simulink model "EVTOLTiltrotor"  (R2024b)
settings: Solver=ode1  StartTime=0.0  StopTime=simTime  RelTol=1e-3  AbsTol=1e-3
undefined symbols (not defined in the file): battery, CityMission, control, FixedWingMission, flightState, FSState, HoverMission, iniRoll, initPitch, iniYaw, params, percWeightGain, position, R_LOOKAHEAD, tiltIni, TransitionMission, uavParam, UAVSampleTime, vIni, Vt, xGround, yGround, zGround
libraries: uavalgslib x7, simulink x4, sharedtransform x2, shared6dof x1, simulink_extras x1, sim3dlib x1, uavsim3dlib x1, uavutilslib x1
(part 1 of 2)
settings Model: DataDictionary=VTOLDynamicsData.sldd  PauseTimes=2  Creator=jjha  LastModifiedBy=jjha
settings SolverCC: AutoInsertRateTranBlk=on  DecoupledContinuousIntegration=on
settings RTWCC: GPUComputeCapability=3.5

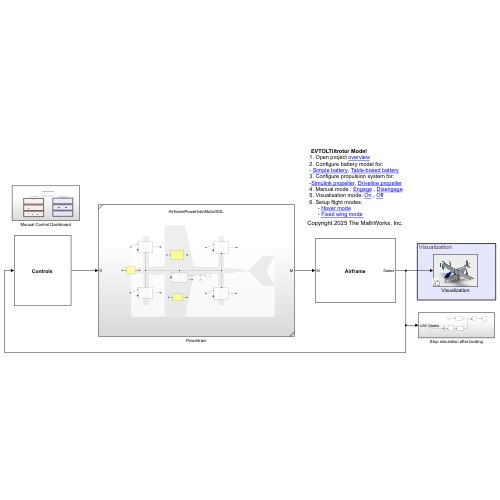
[thumbnail: Simulink's stored preview of the top-level diagram]
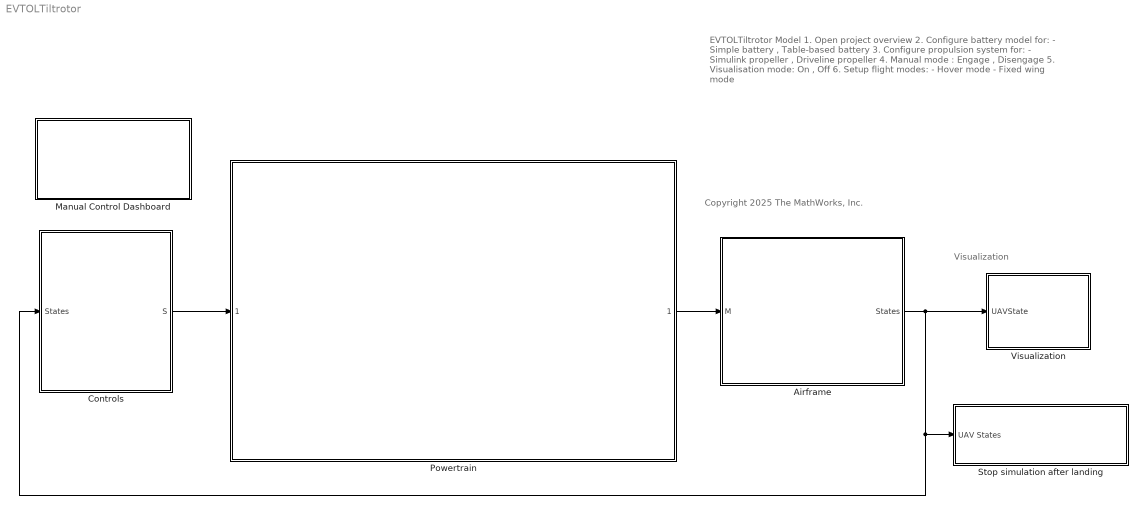
== system EVTOLTiltrotor ==
  note: Copyright 2025 The MathWorks, Inc.
  note: Visualization
  note: EVTOLTiltrotor Model
      | 1. Open project overview
      | 2. Configure battery model for:
      | - Simple battery , Table-based battery
      | 3. Configure propulsion system for:
      | - Simulink propeller , Driveline propeller
      | 4. Manual mode : Engage , Disengage
      | 5. Visualisation mode: On , Off
      | 6. Setup flight modes:
      | - Hover mode
      | - Fixed wing mode
  Airframe : Subsystem
      mask Display:
      | %disp(get_param(gcb, 'Name'))
      | disp(['{\bf\fontsize{12}' get_param(gcb, 'Name') '}'], 'texmode','on');
  Controls : Subsystem
      mask Display:
      | %disp(get_param(gcb, 'Name'))
      | disp(['{\bf\fontsize{12}' get_param(gcb, 'Name') '}'], 'texmode','on');
  Manual Control Dashboard : Subsystem
  Powertrain : Subsystem  ReferencedSubsystem=AirframePowertrainMotorSDL
  Stop simulation after landing : Subsystem
  Visualization : Subsystem  Variant=on  VariantControl=Visualization
      mask Display: image('TiltrotorVisualization.PNG'); % Use "Edit Image" on toolstrip to change.
  wires:
  Controls/1(S) -> Powertrain/1
  Airframe/1(States) -> Controls/1(States), Stop simulation after landing/1(UAV States), Visualization/1(UAVState)
  Powertrain/1 -> Airframe/1(M)

== system EVTOLTiltrotor/Airframe ==
  M : Inport
  6DOF (Euler Angles) : shared6dof/6DOF (Euler Angles)  units=Metric (MKS)  mtype=Fixed  rep=Euler Angles  xme_0=[xGround, yGround, zGround]  Vm_0=[vIni 0 0]  eul_0=[iniRoll initPitch iniYaw]  pm_0=[0 0 0]  mass_0=6.031*percWeightGain  mass_e=0.5  mass_f=2.0  inertia=[uavParam.geom.Ixx 0 0; 0 uavParam.geom.Iyy 0; 0 0 uavParam.geom.Izz]*percWeightGain  inertia_e=eye(3)  inertia_f=2*eye(3)  k_quat=1.0  vre_flag=on  abi_flag=on  aMode=0  xme_statename=''  Vm_statename=''  eul_statename=''  quat_statename=''  pm_statename=''  mass_statename=''
  Energy : Subsystem
      mask Display:
      | %disp(get_param(gcb, 'Name'))
      | disp(['{\bf\fontsize{12}' get_param(gcb, 'Name') '}'], 'texmode','on');
  Ground Truth Bus : Subsystem
  Input : Subsystem
  Scope : Scope  NumInputPorts=2
  Terminator : Terminator
  States : Outport
  wires:
  Input/4(AirData) -> Ground Truth Bus/10(AirData)
  Input/3(RotorPar) -> Ground Truth Bus/9(RotorParams)
  Ground Truth Bus/1(Ground Truth) -> States/1  "States"
  Input/2(M) -> Scope/2, 6DOF (Euler Angles)/2  "Moment"
  Input/1(F) -> Scope/1, 6DOF (Euler Angles)/1  "Thrust"
  6DOF (Euler Angles)/9 -> Ground Truth Bus/8(Abe)
  6DOF (Euler Angles)/7 -> Terminator/1
  6DOF (Euler Angles)/8 -> Ground Truth Bus/7(Abb)  "Abb"
  6DOF (Euler Angles)/5 -> Ground Truth Bus/5(Vb)  "Vb"
  6DOF (Euler Angles)/1 -> Ground Truth Bus/1(Ve)  "Ve"
  6DOF (Euler Angles)/2 -> Ground Truth Bus/2(Xe)  "Xe"
  6DOF (Euler Angles)/4 -> Ground Truth Bus/4(DCMbe)  "DCMbe"
  6DOF (Euler Angles)/3 -> Ground Truth Bus/3(Euler)  "Euler"
  6DOF (Euler Angles)/6 -> Ground Truth Bus/6(pqr)  "pqr"
  M/1 -> Energy/1(s), Input/1(m)

== system EVTOLTiltrotor/Controls ==
  States : Inport
  Bus Creator : BusCreator  Inputs=2
  Constant1 : Constant
  Flight Control : Subsystem  ReferencedSubsystem=FlightControl
      settings: PortSchema="{\"entries\":[{\"content\":{\"sides\":[{\"content\":{\"connectorIds\":[\"In1\",\"In3\",\"In2\"]},\"type\":\"ConnectorPlacement.EquallySpacedRectSide\",\"uuid\":\"16133643-a271-41ca-af0b-35692e75911e\"},{\"content\":{\"connectorIds\":[\"Out1\",\"Out3\",\"Out2\"],\"side\":\"RIGHT\"},\"type\":\"ConnectorPlacement.EquallySpacedRectSide\",\"uuid\":\"71f512ce-dc43-4a94-9ca9-7a68bb7e8691\"},{\"content\":{\"side\":\"TOP\"},\"type\":\"ConnectorPlacement.EquallySpacedRectSide\",\"uuid\":\"92fc6d85-868c-4302-9641-f62c34b61a8f\"}]},\"type\":\"ConnectorPlacement.EquallySpacedConnector\",\"uuid\":\"8e64feec-9c48-46d7-b9b5-e6a25dfded6a\"}],\"packageUris\":[\"http://schema.mathworks.com/mf0/Connector/R2020b\"],\"version\":\"1.0\"}"
  Guidance Test Bench : Subsystem
  Output : Subsystem
  Sensor : Subsystem
  noQGC : Subsystem  TreatAsAtomicUnit=on  SystemSampleTime=UAVSampleTime*4  VariantControl=useQGC==0
  S : Outport
  wires:
  Output/1(S) -> S/1
  Bus Creator/1 -> Output/1(Act)
  Flight Control/3 -> Bus Creator/2  "Tq"
  Flight Control/1 -> Bus Creator/1  "Actuator"
  noQGC/1(Mission) -> Guidance Test Bench/1(Global Mission)
  Guidance Test Bench/1(Cmd) -> Flight Control/1
  States/1 -> Output/3(States), Sensor/1("  "), Guidance Test Bench/2(Aircraft States)
  Flight Control/2 -> Output/2(Ctrl)  "CtrlSurfaces"
  Sensor/1(" ") -> Flight Control/2
  Constant1/1 -> Flight Control/3

== system EVTOLTiltrotor/Manual Control Dashboard ==
  note: Commanded Altitude
  note: Flight Mode
  note: Commanded Y (m)
  note: Fixed Wing
  note: Commanded Airspeed (m)
  note: Hover
  note: Transition
  note: Commanded Course
  note: Fixed Wing Commands
  note: Hover Commands
  note: Commanded Altitude (m)
  note: Back Transition
  note: Commanded X (m)
  note: Change these parameters during simulation when using manual testbench mode. To engage manual testbench mode set variable TestMode=0
  FlightModeSlider : SliderBlock  LabelPosition=Hide  ScaleMax=3  TickInterval=1
  Slider1 : SliderBlock  LabelPosition=Hide  ScaleMax=50  TickInterval=5
  Slider2 : SliderBlock  LabelPosition=Hide  ScaleMin=-30  ScaleMax=30  TickInterval=5
  Slider3 : SliderBlock  LabelPosition=Hide  ScaleMin=-30  ScaleMax=30  TickInterval=5
  Slider5 : SliderBlock  LabelPosition=Hide  ScaleMin=-30  ScaleMax=30  TickInterval=5
  Slider6 : SliderBlock  LabelPosition=Hide  ScaleMin=-100  TickInterval=10
  Slider7 : SliderBlock  LabelPosition=Hide  ScaleMin=10  ScaleMax=30  TickInterval=5

== system EVTOLTiltrotor/Stop simulation after landing ==
  UAV States : Inport
  AND : Logic  IconShape=distinctive  AllPortsSameDT=off  OutDataTypeStr=boolean
  Bus Selector : BusSelector  OutputSignals=Xe
  Clock : Clock
  Compare To Constant : simulink/Logic and Bit Operations/Compare To Constant  relop=>=  const=-1e-1  OutDataTypeStr=boolean
  Compare To Constant1 : simulink/Logic and Bit Operations/Compare To Constant  relop=>=  const=5  OutDataTypeStr=boolean
  Selector : Selector  InputPortWidth=3  IndexOptions=Index vector (dialog)  Indices=3  OutputSizes=1
  Stop Simulation : Stop
  wires:
  Bus Selector/1 -> Selector/1  "<Xe>"
  AND/1 -> Stop Simulation/1
  Compare To Constant1/1 -> AND/1
  UAV States/1 -> Bus Selector/1
  Clock/1 -> Compare To Constant1/1
  Compare To Constant/1 -> AND/2
  Selector/1 -> Compare To Constant/1

== system EVTOLTiltrotor/Visualization ==
  UAVState : Inport
  No Visualization : Subsystem  VariantControl=Visualization==0
  Photorealistic : Subsystem  VariantControl=Visualization==2
  Visualization : Subsystem  VariantControl=Visualization==1

== system EVTOLTiltrotor/Airframe/Energy ==
  note: Range Estimator
  s : Inport
  Add : Sum  Inputs=++++
  Add1 : Sum
  Bus Selector : BusSelector  OutputSignals=R1.Info,R2.Info,R3.Info,R4.Info,A.AirData.airspeed,Batt.Current,Batt.Volt
  Distance : Subsystem
  Energy : Display
  Energy Consumed : Display
  Energy Motor1 : Subsystem
  Energy Motor2 : Subsystem
  Energy Motor3 : Subsystem
  Energy Motor4 : Subsystem
  Online Range : Subsystem
  Range Rating : Subsystem
  Scope : Scope  NumInputPorts=2
  Terminator : Terminator
  Zero division protection : Constant  Value=0.01
  wires:
  Bus Selector/1 -> Energy Motor1/1(M1)  "<Info>"
  Bus Selector/2 -> Energy Motor2/1(M2)  "<Info>"
  Bus Selector/3 -> Energy Motor3/1(M3)  "<Info>"
  Bus Selector/4 -> Energy Motor4/1(M4)  "<Info>"
  Energy Motor2/1(E2) -> Add/2
  Energy Motor3/1(E3) -> Add/3
  Energy Motor4/1(E4) -> Add/4
  Add/1 -> Energy Consumed/1
  Energy Motor1/1(E1) -> Add/1
  Distance/1(Dist) -> Add1/2
  Add1/1 -> Range Rating/1(d)
  Distance/2(SimTime(s)) -> Terminator/1
  Zero division protection/1 -> Add1/1
  Online Range/1(E) -> Range Rating/2(E), Energy/1
  s/1 -> Bus Selector/1
  Bus Selector/5 -> Distance/1(VehSpd)  "<airspeed>"
  Bus Selector/6 -> Scope/1, Online Range/1(I)  "<Current>"
  Bus Selector/7 -> Online Range/2(V), Scope/2  "<Volt>"

== system EVTOLTiltrotor/Airframe/Ground Truth Bus ==
  Ve : Inport
  Xe : Inport  Port=2
  Euler : Inport  Port=3
  DCMbe : Inport  Port=4
  Vb : Inport  Port=5
  pqr : Inport  Port=6
  Abb : Inport  Port=7
  Abe : Inport  Port=8
  RotorParams : Inport  Port=9
  AirData : Inport  Port=10
  Bus Creator : BusCreator  Inputs=13
  Bus Selector : BusSelector  OutputSignals=airspeed
  Direction Cosine Matrix to Quaternions : sharedtransform/Direction Cosine Matrix  to Quaternions  aMode=0  action=None  tolerance=eps(2)
      settings: LibrarySourceBlock=|
      | aerolibtransform2/Direction Cosine Matrix
      | to Quaternions
  Ground Track : MATLAB Function  TreatAsAtomicUnit=on
  To Workspace : ToWorkspace  VariableName=PositionPlotData  SaveFormat=Timeseries  SampleTime=-1
  Ground Truth : Outport
  wires:
  Ve/1 -> Bus Creator/1, Ground Track/1(vxyz)
  Ground Track/1(course) -> Bus Creator/12  "course"
  Ground Track/2(gndSpeed) -> Bus Creator/13  "gndspeed"
  Abe/1 -> Bus Creator/11  "Abe"
  RotorParams/1 -> Bus Creator/8  "RotorParameters"
  Direction Cosine Matrix to Quaternions/1 -> Bus Creator/10  "q"
  Bus Selector/1 -> Bus Creator/9  "<airspeed>"
  AirData/1 -> Bus Selector/1
  Abb/1 -> Bus Creator/7
  Vb/1 -> Bus Creator/5
  Euler/1 -> Bus Creator/3
  DCMbe/1 -> Bus Creator/4, Direction Cosine Matrix to Quaternions/1
  Bus Creator/1 -> Ground Truth/1
  Xe/1 -> To Workspace/1, Bus Creator/2
  pqr/1 -> Bus Creator/6

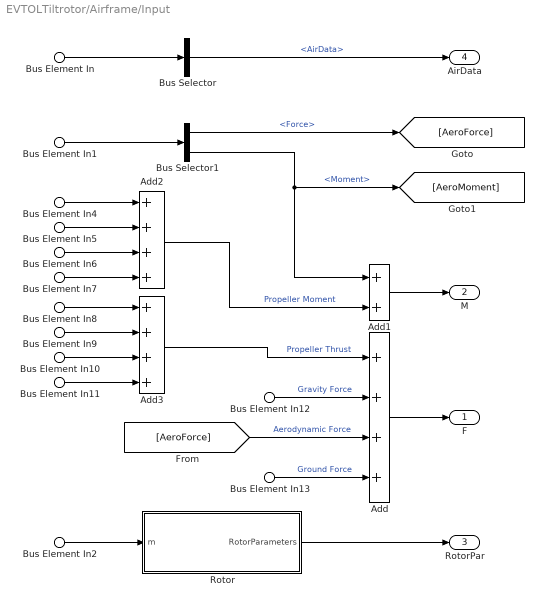
== system EVTOLTiltrotor/Airframe/Input ==
  Bus Element In2 : Inport  PortName=m
  Bus Element In : Inport  PortName=m  Element=A
  Bus Element In1 : Inport  PortName=m  Element=A
  Bus Element In4 : Inport  PortName=m  Element=R1.M
  Bus Element In8 : Inport  PortName=m  Element=R1.F
  Bus Element In5 : Inport  PortName=m  Element=R2.M
  Bus Element In9 : Inport  PortName=m  Element=R2.F
  Bus Element In6 : Inport  PortName=m  Element=R3.M
  Bus Element In10 : Inport  PortName=m  Element=R3.F
  Bus Element In7 : Inport  PortName=m  Element=R4.M
  Bus Element In11 : Inport  PortName=m  Element=R4.F
  Bus Element In12 : Inport  PortName=m  Element=G.gravityForce
  Bus Element In13 : Inport  PortName=m  Element=AD.GroundForce
  Add : Sum  Inputs=++++
  Add1 : Sum
  Add2 : Sum  Inputs=++++
  Add3 : Sum  Inputs=++++
  Bus Selector : BusSelector  OutputSignals=AirData
  Bus Selector1 : BusSelector  OutputSignals=Force,Moment
  Rotor : Subsystem
  F : Outport
  M : Outport  Port=2
  RotorPar : Outport  Port=3
  AirData : Outport  Port=4
  wires:
  Bus Element In12/1 -> Add/2  "Gravity Force"
  Add3/1 -> Add/1  "Propeller Thrust"
  [AeroForce] -> Add/3  "Aerodynamic Force"
  Add2/1 -> Add1/2  "Propeller Moment"
  Add/1 -> F/1
  Bus Element In13/1 -> Add/4  "Ground Force"
  Bus Selector1/1 -> [AeroForce]  "<Force>"
  Add1/1 -> M/1
  Bus Selector1/2 -> Add1/1, [AeroMoment]  "<Moment>"
  Rotor/1(RotorParameters) -> RotorPar/1
  Bus Selector/1 -> AirData/1  "<AirData>"
  Bus Element In/1 -> Bus Selector/1
  Bus Element In1/1 -> Bus Selector1/1
  Bus Element In2/1 -> Rotor/1(m)
  Bus Element In4/1 -> Add2/1
  Bus Element In5/1 -> Add2/2
  Bus Element In6/1 -> Add2/3
  Bus Element In7/1 -> Add2/4
  Bus Element In10/1 -> Add3/3
  Bus Element In8/1 -> Add3/1
  Bus Element In9/1 -> Add3/2
  Bus Element In11/1 -> Add3/4

== system EVTOLTiltrotor/Controls/Guidance Test Bench ==
  Global Mission : Inport
  Aircraft States : Inport  Port=2
  Bus Creator : BusCreator  Inputs=5
  Constant : Constant  Value=0
  ControlType : Subsystem  Variant=on  VariantControl=Choice
  Rate Transition : RateTransition  OutPortSampleTime=0.005
  Variant Subsystem : Subsystem  Variant=on
      settings: PortSchema="{\"entries\":[{\"content\":{\"sides\":[{\"content\":{\"connectorIds\":[\"In1\"]},\"type\":\"ConnectorPlacement.EquallySpacedRectSide\",\"uuid\":\"9fdb7eb7-bc98-4ae8-8dfe-5c3a3cbe5bd4\"},{\"content\":{\"connectorIds\":[\"In2\",\"In3\"],\"side\":\"RIGHT\"},\"type\":\"ConnectorPlacement.EquallySpacedRectSide\",\"uuid\":\"6c20d813-5cc1-435b-898c-bc09e61a7ed0\"},{\"content\":{\"side\":\"TOP\"},\"type\":\"ConnectorPlacement.EquallySpacedRectSide\",\"uuid\":\"a99c14f5-f5c7-4b02-b3e4-43ca7266f03f\"}]},\"type\":\"ConnectorPlacement.EquallySpacedConnector\",\"uuid\":\"e822b786-0a0c-436e-b41c-201e2beca970\"}],\"packageUris\":[\"http://schema.mathworks.com/mf0/Connector/R2020b\"],\"version\":\"1.0\"}"
  Cmd : Outport
  wires:
  Rate Transition/1 -> Variant Subsystem/1(State), ControlType/1(Aircraft States)
  ControlType/3(AACSP) -> Variant Subsystem/3(AAC), Bus Creator/3  "AACSP"
  ControlType/4(ctrlMode) -> Bus Creator/4  "ctrlMode"
  ControlType/5(FlightMode) -> Bus Creator/5  "FlightMode"
  ControlType/2(FixedWingSP) -> Bus Creator/2  "FixedWingSP"
  Global Mission/1 -> ControlType/2(Global Mission)
  ControlType/1(HoverCmds) -> Variant Subsystem/2(Position), Bus Creator/1  "HoverSP"
  Aircraft States/1 -> Rate Transition/1
  Bus Creator/1 -> Cmd/1
  Constant/1 -> ControlType/3(Ground)

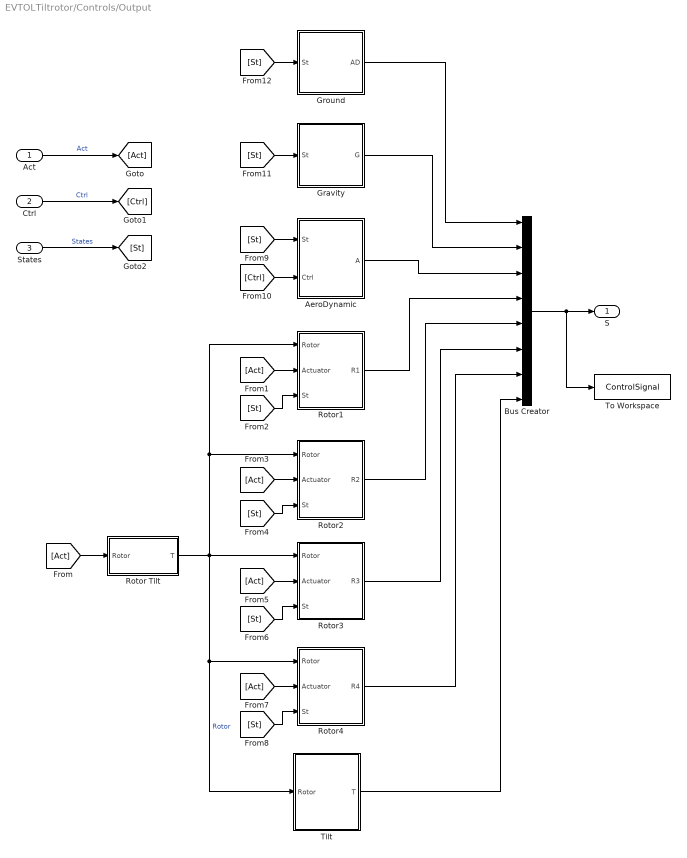
== system EVTOLTiltrotor/Controls/Output ==
  Act : Inport
  Ctrl : Inport  Port=2
  States : Inport  Port=3
  AeroDynamic : Subsystem
  Bus Creator : BusCreator  Inputs=8
  Gravity : Subsystem
  Ground : Subsystem
  Rotor Tilt : Subsystem
  Rotor1 : Subsystem
  Rotor2 : Subsystem
  Rotor3 : Subsystem
  Rotor4 : Subsystem
  Tilt : Subsystem
  To Workspace : ToWorkspace  VariableName=ControlSignal  SaveFormat=Timeseries  SampleTime=-1
  S : Outport
  wires:
  Rotor Tilt/1(T) -> Rotor1/1(Rotor), Rotor2/1(Rotor), Tilt/1(Rotor), Rotor4/1(Rotor), Rotor3/1(Rotor)  "Rotor"
  States/1 -> [St]  "States"
  Act/1 -> [Act]  "Act"
  Ctrl/1 -> [Ctrl]  "Ctrl"
  [Act] -> Rotor Tilt/1(Rotor)
  [Act] -> Rotor1/2(Actuator)
  Rotor1/1(R1) -> Bus Creator/4
  [St] -> Rotor1/3(St)
  [St] -> Rotor2/3(St)
  Rotor2/1(R2) -> Bus Creator/5
  [Act] -> Rotor2/2(Actuator)
  [Act] -> Rotor3/2(Actuator)
  [St] -> Rotor3/3(St)
  [St] -> Rotor4/3(St)
  [Act] -> Rotor4/2(Actuator)
  Rotor3/1(R3) -> Bus Creator/6
  Rotor4/1(R4) -> Bus Creator/7
  [St] -> AeroDynamic/1(St)
  [Ctrl] -> AeroDynamic/2(Ctrl)
  AeroDynamic/1(A) -> Bus Creator/3
  [St] -> Gravity/1(St)
  Gravity/1(G) -> Bus Creator/2
  [St] -> Ground/1(St)
  Ground/1(AD) -> Bus Creator/1
  Tilt/1(T) -> Bus Creator/8
  Bus Creator/1 -> To Workspace/1, S/1

== system EVTOLTiltrotor/Controls/Sensor ==
  "  " : Inport
  No Sensors Dynamics : Subsystem  VariantControl=SensorType==0
  Rate Transition : RateTransition  OutPortSampleTime=0.005
  " " : Outport
  wires:
  No Sensors Dynamics/1(SensorData) -> " "/1
  "  "/1 -> No Sensors Dynamics/1(UAVStates)

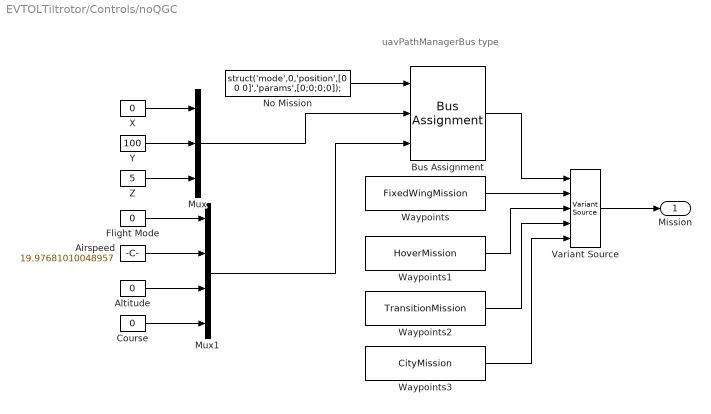
== system EVTOLTiltrotor/Controls/noQGC ==
  note: uavPathManagerBus type
  Airspeed : Constant  Value=19.97681010048957
  Altitude : Constant  Value=0
  Bus Assignment : BusAssignment  AssignedSignals=position,params
  Course : Constant  Value=0
  Flight Mode : Constant  Value=0
  Mux : Mux  Inputs=3
  Mux1 : Mux
  No Mission : Constant  Value=struct('mode',0,'position',[0 0 0]','params',[0;0;0;0]);  OutDataTypeStr=Bus: doubleUavPathManager
  Variant Source : VariantSource
  Waypoints : Constant  Value=FixedWingMission  OutDataTypeStr=Bus: doubleUavPathManager  SampleTime=-1
  Waypoints1 : Constant  Value=HoverMission  OutDataTypeStr=Bus: doubleUavPathManager  SampleTime=-1
  Waypoints2 : Constant  Value=TransitionMission  OutDataTypeStr=Bus: doubleUavPathManager  SampleTime=-1
  Waypoints3 : Constant  Value=CityMission  OutDataTypeStr=Bus: doubleUavPathManager  SampleTime=-1
  X : Constant  Value=0
  Y : Constant  Value=100
  Z : Constant  Value=5
  Mission : Outport
  wires:
  Waypoints/1 -> Variant Source/2
  Waypoints1/1 -> Variant Source/3
  Variant Source/1 -> Mission/1
  Waypoints2/1 -> Variant Source/4
  No Mission/1 -> Bus Assignment/1
  Waypoints3/1 -> Variant Source/5
  Bus Assignment/1 -> Variant Source/1
  X/1 -> Mux/1
  Y/1 -> Mux/2
  Z/1 -> Mux/3
  Mux/1 -> Bus Assignment/2
  Mux1/1 -> Bus Assignment/3
  Flight Mode/1 -> Mux1/1
  Course/1 -> Mux1/4
  Altitude/1 -> Mux1/3
  Airspeed/1 -> Mux1/2

== system EVTOLTiltrotor/Visualization/No Visualization ==
  UAVState : Inport
  Terminator : Terminator
  wires:
  UAVState/1 -> Terminator/1

== system EVTOLTiltrotor/Visualization/Photorealistic ==
  UAVState : Inport
  Bus Creator : BusCreator  Inputs=6
  Bus Selector : BusSelector  OutputSignals=Euler,Xe
  Demux : Demux  Outputs=3
  Demux1 : Demux  Outputs=3
  Prepare UAV Data : Subsystem
  Simulation 3D Scene Configuration : sim3dlib/Simulation 3D Scene Configuration  Priority=0  ProjectFormat=Unreal Editor  SceneDesc=US city block  ProjectName=I:\29\vdubey.MergedFixedWingReview\matlab\toolbox\shared\sim3d_projects\automotive_project_windows\UE\WindowsNoEditor\VehicleSimulation.exe  ScenePath=/Game/Maps/USCityBlock  UEProjPath=C:\Documents\project\AutoVrtlEnv\AutoVrtlEnv.uproject  EnableOpenDRIVE=off  vehTagList={'Custom';'Scene Origin';'VTOL_Vehicle'}  vehTag=VTOL_Vehicle  FreeCameraInitialTranslation=[0, 0, 0]  FreeCameraDefaultInitialTranslation=[-6, 0, 2]  FreeCameraInitialRotation=[0, 0, 0]  FreeCameraDefaultInitialRotation=[0, -15, 0]  OpVisEn=off  Ts=1/10  EnableWindow=on  EnableRemoteAccess=off  EnableWeather=off  SunAzimuth=90  SunAltitude=40.0  EnableGeospatialSun=off  Latitude=0  Longitude=0  Date=2023-01-01  Time=10:30:00  GeoTimeZone=-5.0  SunDaylightSaving=off  wind=1  clouds=10  EnableVolumetricClouds=off  CloudCoverage=0  CloudAltitude=6  fog=0  rain=0  RaindropsEffect=off  SnowDensity=0  EnableGeospatial=off  UseTrueOrigin=off  OriginHeight=200  OriginLatitude=40.744652  OriginLongitude=-73.988864  MapStyle=Aerial  AdditionalAssetIDs=[]  UseAdvancedSunSky=off  SolarTime=11  TimeZone=-5  Day=21  Month=9  Year=2022  UseDaylightSavingTime=on  DSTStartDay=10  DSTStartMonth=3  DSTEndDay=3  DSTEndMonth=11  DSTSwitchHour=2  sensorTag=MainCamera2  sensorId=2  sensorName=MainCamera2  mountLoc=Origin  offsetFlag=off  tmountOffset=[0, 0, 0]  rmountOffset=[0, 0, 0]  HorizontalResolution=1280  VerticalResolution=720  HorizontalFOV=60  mountPoint=[0 0 0]  mountOrientation=[0 0 0]  aMode=4  ID=2  GeoTrigger=Inactive
      settings: LibrarySourceBlock=uavsim3dlib/Simulation 3D Scene Configuration
  Simulation 3D UAV Vehicle : uavsim3dlib/Simulation 3D UAV Vehicle  Priority=-1  Mesh=Custom  MeshPath=SkeletalMesh'/Game/Maps/VTOLDEMO/VTOLAsset.VTOLAsset'  Color=Black  ActorName=VTOL_Vehicle  UseGlobalFrame=off  InitialTranslation=[0 0 0]  InitialRotation=[0 0 0]  InitialTranslationGlobal=[0 0 0]  InitialGeoOrigin=[0 0 0]  InitialRotationGlobal=[0 0 0]  SampleTime=0.1  ActorType=SimulinkVehicle  ID=C  aMode=4  ActorTag=VTOL_Vehicle
  wires:
  UAVState/1 -> Bus Selector/1
  Bus Selector/2 -> Demux1/1  "<Xe>"
  Bus Selector/1 -> Demux/1  "<Euler>"
  Prepare UAV Data/2(Rotation) -> Simulation 3D UAV Vehicle/2
  Demux/1 -> Bus Creator/1  "roll"
  Demux/3 -> Bus Creator/3  "yaw"
  Demux1/1 -> Bus Creator/4  "x"
  Demux1/2 -> Bus Creator/5  "y"
  Bus Creator/1 -> Prepare UAV Data/1(UAVState)
  Demux1/3 -> Bus Creator/6  "z"
  Demux/2 -> Bus Creator/2  "pitch"
  Prepare UAV Data/1(Translation) -> Simulation 3D UAV Vehicle/1

== system EVTOLTiltrotor/Visualization/Visualization ==
  UAVState : Inport
  Bus Selector : BusSelector  OutputSignals=Xe,q,RotorParameters.Tilt1,RotorParameters.Tilt2
  Gain : Gain  Gain=0
  Subsystem : Subsystem
  Trajectory : uavutilslib/UAV Animation  NumUAV=1  DynamicUAVConfig=off  UAVType=FixedWing  UAVSize=5  UAVColor=[1 0 0]  UAVTrajectoryAlpha=1  InertialZDirection=Down  RotationFormat=Quaternion  DrawMarkers=off  SampleTime=0.1
  wires:
  Bus Selector/2 -> Subsystem/2(<q>), Trajectory/2  "<q>"
  Bus Selector/1 -> Trajectory/1, Gain/1  "<Xe>"
  Gain/1 -> Subsystem/1(<Xe>)
  UAVState/1 -> Bus Selector/1
  Bus Selector/3 -> Subsystem/3(RotorA)  "<Tilt1>"
  Bus Selector/4 -> Subsystem/4(RotorB)  "<Tilt2>"

== system EVTOLTiltrotor/Airframe/Energy/Distance ==
  VehSpd : Inport
  Add : Sum
  Constant : Constant
  Constant1 : Constant  Value=0.1
  Display : Display
  Divide : Product  Inputs=*/
  Integrator : Integrator
  Integrator1 : Integrator
  Dist : Outport
  SimTime(s) : Outport  Port=2
  wires:
  Divide/1 -> Display/1
  Integrator/1 -> Dist/1, Divide/1  "Distance"
  VehSpd/1 -> Integrator/1
  Add/1 -> SimTime(s)/1, Divide/2
  Integrator1/1 -> Add/1  "time"
  Constant1/1 -> Add/2
  Constant/1 -> Integrator1/1

== system EVTOLTiltrotor/Airframe/Energy/Energy Motor1 ==
  Bus Element In : Inport  PortName=M1  Element=Current
  Bus Element In1 : Inport  PortName=M1  Element=Volt
  Integrator : Integrator
  Product : Product
  E1 : Outport
  wires:
  Bus Element In/1 -> Product/1
  Bus Element In1/1 -> Product/2
  Product/1 -> Integrator/1
  Integrator/1 -> E1/1

== system EVTOLTiltrotor/Airframe/Energy/Energy Motor2 ==
  Bus Element In : Inport  PortName=M2  Element=Current
  Bus Element In1 : Inport  PortName=M2  Element=Volt
  Integrator : Integrator
  Product : Product
  E2 : Outport
  wires:
  Integrator/1 -> E2/1
  Product/1 -> Integrator/1
  Bus Element In1/1 -> Product/2
  Bus Element In/1 -> Product/1

== system EVTOLTiltrotor/Airframe/Energy/Energy Motor3 ==
  Bus Element In : Inport  PortName=M3  Element=Current
  Bus Element In1 : Inport  PortName=M3  Element=Volt
  Integrator : Integrator
  Product : Product
  E3 : Outport
  wires:
  Bus Element In/1 -> Product/1
  Bus Element In1/1 -> Product/2
  Product/1 -> Integrator/1
  Integrator/1 -> E3/1

== system EVTOLTiltrotor/Airframe/Energy/Energy Motor4 ==
  Bus Element In : Inport  PortName=M4  Element=Current
  Bus Element In1 : Inport  PortName=M4  Element=Volt
  Integrator : Integrator
  Product : Product
  E4 : Outport
  wires:
  Integrator/1 -> E4/1
  Product/1 -> Integrator/1
  Bus Element In1/1 -> Product/2
  Bus Element In/1 -> Product/1

== system EVTOLTiltrotor/Airframe/Energy/Online Range ==
  note: Total energy consumed
  note: Energy Consumption
  I : Inport
  V : Inport  Port=2
  Abs : Abs  SaturateOnIntegerOverflow=off
  Constant : Constant  Value=3600
  Divide : Product  Inputs=*/
  Integrator : Integrator
  Product : Product
  To Workspace : ToWorkspace  VariableName=elecPower  SaveFormat=Timeseries  SampleTime=-1
  E : Outport
  wires:
  Divide/1 -> E/1  "Energy"
  Abs/1 -> Product/2
  Constant/1 -> Divide/2
  Integrator/1 -> Divide/1
  Product/1 -> To Workspace/1, Integrator/1
  V/1 -> Product/1
  I/1 -> Abs/1

== system EVTOLTiltrotor/Airframe/Energy/Range Rating ==
  note: Energy consumption rate = Total energy consumed / Total flight distance
      | Range = Energy in battery / Energy consumption rate
  note: Total capacity at full charge , Ahr*BatVoltage*CellinSeries
  d : Inport
  E : Inport  Port=2
  Add : Sum
  Constant : Constant  Value=eps
  Display : Display
  Divide : Product  Inputs=*/
  Divide1 : Product  Inputs=/*
  To Workspace : ToWorkspace  VariableName=EnergyMileage  SaveFormat=Timeseries  SampleTime=-1
  TotalEnergy : Constant  Value=battery.AH*battery.Np
  wires:
  TotalEnergy/1 -> Divide1/2
  Divide/1 -> To Workspace/1, Add/2
  Divide1/1 -> Display/1  "RangeRating"
  d/1 -> Divide/2
  E/1 -> Divide/1
  Constant/1 -> Add/1
  Add/1 -> Divide1/1

== system EVTOLTiltrotor/Airframe/Input/Rotor ==
  Bus Element In : Inport  PortName=m  Element=R1.W
  Bus Element In4 : Inport  PortName=m  Element=R1.T
  Bus Element In10 : Inport  PortName=m  Element=R1.Tilt
  Bus Element In1 : Inport  PortName=m  Element=R2.W
  Bus Element In5 : Inport  PortName=m  Element=R2.T
  Bus Element In11 : Inport  PortName=m  Element=R2.Tilt
  Bus Element In2 : Inport  PortName=m  Element=R3.W
  Bus Element In6 : Inport  PortName=m  Element=R3.T
  Bus Element In3 : Inport  PortName=m  Element=R4.W
  Bus Element In7 : Inport  PortName=m  Element=R4.T
  Bus Creator : BusCreator  Inputs=10
  RotorParameters : Outport
  wires:
  Bus Creator/1 -> RotorParameters/1
  Bus Element In4/1 -> Bus Creator/7  "T1"
  Bus Element In5/1 -> Bus Creator/8  "T2"
  Bus Element In6/1 -> Bus Creator/9  "T3"
  Bus Element In7/1 -> Bus Creator/10  "T4"
  Bus Element In10/1 -> Bus Creator/5  "Tilt1"
  Bus Element In11/1 -> Bus Creator/6  "Tilt2"
  Bus Element In3/1 -> Bus Creator/4  "w4"
  Bus Element In2/1 -> Bus Creator/3  "w3"
  Bus Element In1/1 -> Bus Creator/2  "w2"
  Bus Element In/1 -> Bus Creator/1  "w1"

== system EVTOLTiltrotor/Controls/Guidance Test Bench/ControlType ==
  Aircraft States : Inport
  Global Mission : Inport  Port=2
  Ground : Inport  Port=3
  Guidance Testbench : Subsystem  TreatAsAtomicUnit=on  VariantControl=TestMode==1
  Manual Control : Subsystem  TreatAsAtomicUnit=on  VariantControl=TestMode==0
  HoverCmds : Outport
  FixedWingSP : Outport  Port=2
  AACSP : Outport  Port=3
  ctrlMode : Outport  Port=4
  FlightMode : Outport  Port=5

== system EVTOLTiltrotor/Controls/Guidance Test Bench/Variant Subsystem ==
  note: 1) Add Subsystem or Model blocks as valid variant choices.
      | 2) You cannot connect blocks at this level. At simulation, connectivity is automatically
      | determined, based on the active variant and port name matching.
  State : Inport
  Position : Inport  Port=2
  AAC : Inport  Port=3
  No-op : Subsystem  VariantControl=Deployment == true
  "Reference Tracking " : Subsystem  VariantControl=Deployment == false

== system EVTOLTiltrotor/Controls/Output/AeroDynamic ==
  St : Inport
  Ctrl : Inport  Port=2
  Bus Creator : BusCreator  Inputs=2
  A : Outport
  wires:
  St/1 -> Bus Creator/1  "St"
  Bus Creator/1 -> A/1  "A"
  Ctrl/1 -> Bus Creator/2  "Ctrl"

== system EVTOLTiltrotor/Controls/Output/Gravity ==
  St : Inport
  Bus Creator : BusCreator  Inputs=1
  Bus Selector : BusSelector  OutputSignals=DCMbe
  G : Outport
  wires:
  Bus Selector/1 -> Bus Creator/1  "<DCMbe>"
  St/1 -> Bus Selector/1  "St"
  Bus Creator/1 -> G/1  "G"

== system EVTOLTiltrotor/Controls/Output/Ground ==
  St : Inport
  Bus Creator : BusCreator  Inputs=3
  Bus Selector : BusSelector  OutputSignals=DCMbe,Ve,Xe
  AD : Outport
  wires:
  Bus Creator/1 -> AD/1  "AD"
  St/1 -> Bus Selector/1  "St"
  Bus Selector/1 -> Bus Creator/1  "<DCMbe>"
  Bus Selector/2 -> Bus Creator/2  "<Ve>"
  Bus Selector/3 -> Bus Creator/3  "<Xe>"

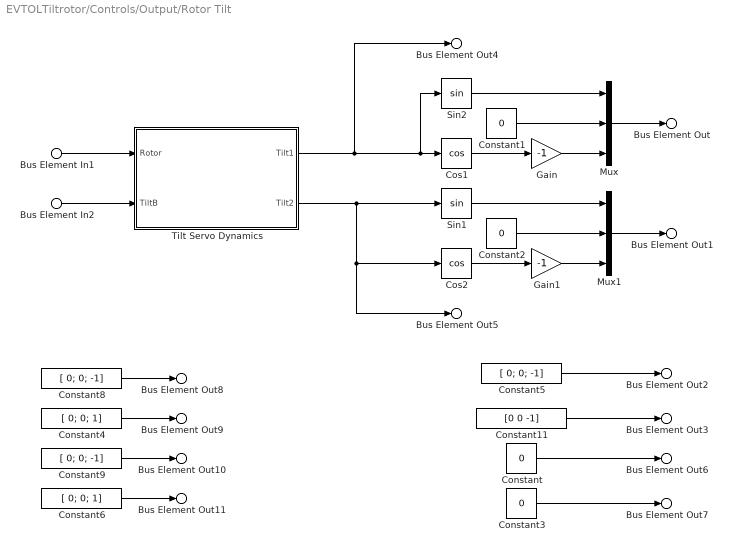
== system EVTOLTiltrotor/Controls/Output/Rotor Tilt ==
  Bus Element In1 : Inport  PortName=Rotor  Element=Actuator.Tilt1
  Bus Element In2 : Inport  PortName=Rotor  Element=Actuator.Tilt2
  Constant{,1..3} (4 alike) : Constant  Value=0
  Constant11 : Constant  Value=[0 0 -1]
  Constant4 : Constant  Value=[ 0; 0; 1]
  Constant5 : Constant  Value=[ 0; 0; -1]
  Constant6 : Constant  Value=[ 0; 0; 1]
  Constant8 : Constant  Value=[ 0; 0; -1]
  Constant9 : Constant  Value=[ 0; 0; -1]
  Cos1 : Trigonometry  Operator=cos
  Cos2 : Trigonometry  Operator=cos
  Gain : Gain  Gain=-1
  Gain1 : Gain  Gain=-1
  Mux : Mux  Inputs=3
  Mux1 : Mux  Inputs=3
  Sin1 : Trigonometry
  Sin2 : Trigonometry
  Tilt Servo Dynamics : Subsystem
  Bus Element Out : Outport  PortName=T  Element=Turn1
  Bus Element Out1 : Outport  PortName=T  Element=Turn2
  Bus Element Out2 : Outport  PortName=T  Element=Turn3
  Bus Element Out3 : Outport  PortName=T  Element=Turn4
  Bus Element Out4 : Outport  PortName=T  Element=Tilt1
  Bus Element Out5 : Outport  PortName=T  Element=Tilt2
  Bus Element Out6 : Outport  PortName=T  Element=Tilt3
  Bus Element Out7 : Outport  PortName=T  Element=Tilt4
  Bus Element Out8 : Outport  PortName=T  Element=Dir1
  Bus Element Out9 : Outport  PortName=T  Element=Dir2
  Bus Element Out10 : Outport  PortName=T  Element=Dir3
  Bus Element Out11 : Outport  PortName=T  Element=Dir4
  wires:
  Constant11/1 -> Bus Element Out3/1
  Mux/1 -> Bus Element Out/1
  Constant1/1 -> Mux/2
  Bus Element In2/1 -> Tilt Servo Dynamics/2(TiltB)
  Bus Element In1/1 -> Tilt Servo Dynamics/1(Rotor)
  Gain/1 -> Mux/3
  Sin2/1 -> Mux/1
  Tilt Servo Dynamics/1(Tilt1) -> Bus Element Out4/1, Sin2/1, Cos1/1
  Mux1/1 -> Bus Element Out1/1
  Gain1/1 -> Mux1/3
  Tilt Servo Dynamics/2(Tilt2) -> Bus Element Out5/1, Cos2/1, Sin1/1
  Sin1/1 -> Mux1/1
  Cos2/1 -> Gain1/1
  Constant2/1 -> Mux1/2
  Cos1/1 -> Gain/1
  Constant5/1 -> Bus Element Out2/1
  Constant/1 -> Bus Element Out6/1
  Constant3/1 -> Bus Element Out7/1
  Constant8/1 -> Bus Element Out8/1
  Constant4/1 -> Bus Element Out9/1
  Constant9/1 -> Bus Element Out10/1
  Constant6/1 -> Bus Element Out11/1

== system EVTOLTiltrotor/Controls/Output/Rotor1 ==
  Rotor : Inport
  Actuator : Inport  Port=2
  St : Inport  Port=3
  Bus Creator : BusCreator  Inputs=2
  Bus Creator1 : BusCreator  Inputs=2
  Bus Creator2 : BusCreator  Inputs=5
  Bus Selector : BusSelector  OutputSignals=Tq.T1,Actuator.w1
  Bus Selector1 : BusSelector  OutputSignals=Turn1,Tilt1,Dir1
  Bus Selector2 : BusSelector  OutputSignals=Vb,pqr
  Gain{,1..4} (5 alike) : Gain
  R1 : Outport
  wires:
  Bus Selector/2 -> Gain/1  "<w1>"
  Bus Selector/1 -> Gain1/1  "<T1>"
  Bus Creator2/1 -> R1/1  "R1"
  Gain/1 -> Bus Creator/2  "Wref"
  Gain1/1 -> Bus Creator/1  "T"
  Rotor/1 -> Bus Selector1/1
  Bus Selector1/1 -> Gain3/1  "<Turn1>"
  Actuator/1 -> Bus Selector/1
  St/1 -> Bus Selector2/1
  Bus Selector2/1 -> Bus Creator1/1  "<Vb>"
  Bus Selector2/2 -> Bus Creator1/2  "<pqr>"
  Bus Creator/1 -> Bus Creator2/1  "Act"
  Bus Creator1/1 -> Bus Creator2/2  "St"
  Gain3/1 -> Bus Creator2/3  "Turn"
  Bus Selector1/2 -> Gain2/1  "<Tilt1>"
  Gain2/1 -> Bus Creator2/4  "Tilt"
  Bus Selector1/3 -> Gain4/1  "<Dir1>"
  Gain4/1 -> Bus Creator2/5  "Dir"

== system EVTOLTiltrotor/Controls/Output/Rotor2 ==
  Rotor : Inport
  Actuator : Inport  Port=2
  St : Inport  Port=3
  Bus Creator : BusCreator  Inputs=2
  Bus Creator1 : BusCreator  Inputs=2
  Bus Creator2 : BusCreator  Inputs=5
  Bus Selector : BusSelector  OutputSignals=Actuator.w2,Tq.T2
  Bus Selector1 : BusSelector  OutputSignals=Turn2,Tilt2,Dir2
  Bus Selector2 : BusSelector  OutputSignals=Vb,pqr
  Gain{,1..4} (5 alike) : Gain
  R2 : Outport
  wires:
  Bus Creator1/1 -> Bus Creator2/2  "St"
  Bus Creator/1 -> Bus Creator2/1  "Act"
  Bus Selector2/2 -> Bus Creator1/2  "<pqr>"
  Bus Selector2/1 -> Bus Creator1/1  "<Vb>"
  St/1 -> Bus Selector2/1
  Actuator/1 -> Bus Selector/1
  Gain1/1 -> Bus Creator/1  "Wref"
  Gain/1 -> Bus Creator/2  "T"
  Bus Creator2/1 -> R2/1  "R2"
  Bus Selector/1 -> Gain1/1  "<w2>"
  Bus Selector/2 -> Gain/1  "<T2>"
  Gain2/1 -> Bus Creator2/4  "Tilt"
  Bus Selector1/2 -> Gain2/1  "<Tilt2>"
  Rotor/1 -> Bus Selector1/1
  Gain3/1 -> Bus Creator2/3  "Turn"
  Bus Selector1/1 -> Gain3/1  "<Turn2>"
  Bus Selector1/3 -> Gain4/1  "<Dir2>"
  Gain4/1 -> Bus Creator2/5  "Dir"

== system EVTOLTiltrotor/Controls/Output/Rotor3 ==
  Rotor : Inport
  Actuator : Inport  Port=2
  St : Inport  Port=3
  Bus Creator : BusCreator  Inputs=2
  Bus Creator1 : BusCreator  Inputs=2
  Bus Creator2 : BusCreator  Inputs=5
  Bus Selector : BusSelector  OutputSignals=Actuator.w3,Tq.T3
  Bus Selector1 : BusSelector  OutputSignals=Turn3,Tilt3,Dir3
  Bus Selector2 : BusSelector  OutputSignals=Vb,pqr
  Gain{,1..4} (5 alike) : Gain
  R3 : Outport
  wires:
  Bus Selector/2 -> Gain/1  "<T3>"
  Bus Selector/1 -> Gain1/1  "<w3>"
  Bus Creator2/1 -> R3/1  "R3"
  Gain/1 -> Bus Creator/2  "T"
  Gain1/1 -> Bus Creator/1  "Wref"
  Actuator/1 -> Bus Selector/1
  St/1 -> Bus Selector2/1
  Bus Selector2/1 -> Bus Creator1/1  "<Vb>"
  Bus Selector2/2 -> Bus Creator1/2  "<pqr>"
  Bus Creator/1 -> Bus Creator2/1  "Act"
  Bus Creator1/1 -> Bus Creator2/2  "St"
  Bus Selector1/1 -> Gain3/1  "<Turn3>"
  Rotor/1 -> Bus Selector1/1
  Gain2/1 -> Bus Creator2/4  "Tilt"
  Bus Selector1/2 -> Gain2/1  "<Tilt3>"
  Gain3/1 -> Bus Creator2/3  "Turn"
  Bus Selector1/3 -> Gain4/1  "<Dir3>"
  Gain4/1 -> Bus Creator2/5  "Dir"

== system EVTOLTiltrotor/Controls/Output/Rotor4 ==
  Rotor : Inport
  Actuator : Inport  Port=2
  St : Inport  Port=3
  Bus Creator : BusCreator  Inputs=2
  Bus Creator1 : BusCreator  Inputs=2
  Bus Creator2 : BusCreator  Inputs=5
  Bus Selector : BusSelector  OutputSignals=Actuator.w4,Tq.T4
  Bus Selector1 : BusSelector  OutputSignals=Turn4,Tilt4,Dir4
  Bus Selector2 : BusSelector  OutputSignals=Vb,pqr
  Gain{,1..4} (5 alike) : Gain
  R4 : Outport
  wires:
  Bus Creator1/1 -> Bus Creator2/2  "St"
  Bus Creator/1 -> Bus Creator2/1  "Act"
  Bus Selector2/2 -> Bus Creator1/2  "<pqr>"
  Bus Selector2/1 -> Bus Creator1/1  "<Vb>"
  St/1 -> Bus Selector2/1
  Actuator/1 -> Bus Selector/1
  Gain1/1 -> Bus Creator/1  "Wref"
  Gain/1 -> Bus Creator/2  "T"
  Bus Creator2/1 -> R4/1  "R4"
  Bus Selector/1 -> Gain1/1  "<w4>"
  Bus Selector/2 -> Gain/1  "<T4>"
  Bus Selector1/1 -> Gain3/1  "<Turn4>"
  Rotor/1 -> Bus Selector1/1
  Gain2/1 -> Bus Creator2/4  "Tilt"
  Bus Selector1/2 -> Gain2/1  "<Tilt4>"
  Gain3/1 -> Bus Creator2/3  "Turn"
  Bus Selector1/3 -> Gain4/1  "<Dir4>"
  Gain4/1 -> Bus Creator2/5  "Dir"

== system EVTOLTiltrotor/Controls/Output/Tilt ==
  Rotor : Inport
  Bus Creator2 : BusCreator  Inputs=2
  Bus Selector1 : BusSelector  OutputSignals=Tilt1,Tilt2
  T : Outport
  wires:
  Bus Creator2/1 -> T/1  "Tilt"
  Rotor/1 -> Bus Selector1/1
  Bus Selector1/1 -> Bus Creator2/1  "<Tilt1>"
  Bus Selector1/2 -> Bus Creator2/2  "<Tilt2>"

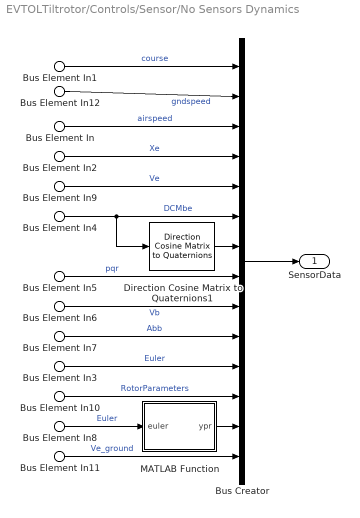
== system EVTOLTiltrotor/Controls/Sensor/No Sensors Dynamics ==
  Bus Element In9 : Inport  PortName=UAVStates  Element=Ve
  Bus Element In11 : Inport  PortName=UAVStates  Element=Ve
  Bus Element In2 : Inport  PortName=UAVStates  Element=Xe
  Bus Element In3 : Inport  PortName=UAVStates  Element=Euler
  Bus Element In8 : Inport  PortName=UAVStates  Element=Euler
  Bus Element In4 : Inport  PortName=UAVStates  Element=DCMbe
  Bus Element In5 : Inport  PortName=UAVStates  Element=pqr
  Bus Element In6 : Inport  PortName=UAVStates  Element=Vb
  Bus Element In7 : Inport  PortName=UAVStates  Element=Abb
  Bus Element In10 : Inport  PortName=UAVStates  Element=RotorParameters
  Bus Element In : Inport  PortName=UAVStates  Element=airspeed
  Bus Element In12 : Inport  PortName=UAVStates  Element=gndspeed
  Bus Element In1 : Inport  PortName=UAVStates  Element=course
  Bus Creator : BusCreator  Inputs=14
  Direction Cosine Matrix to Quaternions1 : sharedtransform/Direction Cosine Matrix  to Quaternions  aMode=0  action=None  tolerance=eps(2)
      settings: LibrarySourceBlock=|
      | aerolibtransform2/Direction Cosine Matrix
      | to Quaternions
  MATLAB Function : MATLAB Function  TreatAsAtomicUnit=on
  SensorData : Outport
  wires:
  Bus Element In1/1 -> Bus Creator/1  "course"
  Bus Element In12/1 -> Bus Creator/2  "gndspeed"
  Bus Element In11/1 -> Bus Creator/14  "Ve_ground"
  Bus Element In3/1 -> Bus Creator/11  "Euler"
  Bus Element In10/1 -> Bus Creator/12  "RotorParameters"
  Bus Element In7/1 -> Bus Creator/10  "Abb"
  Bus Element In6/1 -> Bus Creator/9  "Vb"
  Direction Cosine Matrix to Quaternions1/1 -> Bus Creator/7
  Bus Element In4/1 -> Direction Cosine Matrix to Quaternions1/1, Bus Creator/6  "DCMbe"
  Bus Element In/1 -> Bus Creator/3  "airspeed"
  Bus Element In9/1 -> Bus Creator/5  "Ve"
  MATLAB Function/1(ypr) -> Bus Creator/13
  Bus Element In2/1 -> Bus Creator/4  "Xe"
  Bus Element In5/1 -> Bus Creator/8  "pqr"
  Bus Creator/1 -> SensorData/1
  Bus Element In8/1 -> MATLAB Function/1(euler)  "Euler"

== system EVTOLTiltrotor/Visualization/Photorealistic/Prepare UAV Data ==
  UAVState : Inport
  Bus Selector1 : BusSelector  OutputSignals=x,y,z,yaw,pitch,roll
  Gain{,1..3} (4 alike) : Gain  Gain=-1
  Mux : Mux  Inputs=3
  Mux1 : Mux  Inputs=3
  Translation : Outport
  Rotation : Outport  Port=2
  wires:
  UAVState/1 -> Bus Selector1/1
  Mux/1 -> Translation/1
  Mux1/1 -> Rotation/1  "EulerZYX"
  Bus Selector1/4 -> Gain3/1  "<yaw>"
  Bus Selector1/5 -> Gain2/1  "<pitch>"
  Bus Selector1/6 -> Mux1/3  "<roll>"
  Bus Selector1/3 -> Gain/1  "<z>"
  Bus Selector1/2 -> Gain1/1  "<y>"
  Bus Selector1/1 -> Mux/1  "<x>"
  Gain/1 -> Mux/3
  Gain1/1 -> Mux/2
  Gain2/1 -> Mux1/2
  Gain3/1 -> Mux1/1

== system EVTOLTiltrotor/Visualization/Visualization/Subsystem ==
  <Xe> : Inport
  <q> : Inport  Port=2
  RotorA : Inport  Port=3
  RotorB : Inport  Port=4
  Constant : Constant  Value=0
  Constant1 : Constant  Value=0
  Gain : Gain  Gain=0
  Gain1 : Gain  Gain=-1
  Gain2 : Gain  Gain=-1
  MATLAB System : MATLABSystem  System=exampleHelperTiltRotorAnimator  SampleTime=0.05
      mask Type: exampleHelperTiltRotorAnimator
      mask Display:
      | disp('exampleHelperTiltRotorAnimator');
      | port_label('input',1,'position');
      | port_label('input',2,'orientation');
      | port_label('input',3,'rotorAngles');
  Mux : Mux
  Reshape : Reshape  OutputDimensionality=Customize  OutputDimensions=[1,4]
  Reshape1 : Reshape  OutputDimensionality=Customize  OutputDimensions=[1,4]
  Reshape2 : Reshape  OutputDimensionality=Customize  OutputDimensions=[1,3]
  wires:
  Gain1/1 -> Mux/1
  Constant1/1 -> Mux/4
  Gain2/1 -> Mux/2
  Reshape1/1 -> MATLAB System/3
  Mux/1 -> Reshape1/1
  RotorA/1 -> Gain1/1
  <Xe>/1 -> Gain/1
  Constant/1 -> Mux/3
  RotorB/1 -> Gain2/1
  <q>/1 -> Reshape/1
  Reshape2/1 -> MATLAB System/1
  Reshape/1 -> MATLAB System/2
  Gain/1 -> Reshape2/1

== system EVTOLTiltrotor/Controls/Guidance Test Bench/ControlType/Guidance Testbench ==
  Global Mission : Inport
  Aircraft States : Inport  Port=2
  Ground : Inport  Port=3
  Control Rate Transition : Subsystem
  Guidance Logic : Subsystem  VariantControl=guidanceType==1
  HoverCmds : Outport
  FixedWingSP : Outport  Port=2
  AACSP : Outport  Port=3
  ctrlMode : Outport  Port=4
  FlightMode : Outport  Port=5
  wires:
  Aircraft States/1 -> Guidance Logic/1(UAVState)
  Global Mission/1 -> Guidance Logic/2(GCSCommands)
  Guidance Logic/1(HoverGuidance) -> Control Rate Transition/1("1 ")
  Guidance Logic/2(FixedWingSP) -> Control Rate Transition/2(In2)
  Guidance Logic/3(AACSP) -> Control Rate Transition/3(In3)
  Guidance Logic/4(ctrlMode) -> Control Rate Transition/4(In4)
  Guidance Logic/5(FlightMode) -> Control Rate Transition/5(In5)
  Control Rate Transition/1(Out1) -> HoverCmds/1
  Control Rate Transition/2(Out2) -> FixedWingSP/1
  Control Rate Transition/3(Out3) -> AACSP/1
  Control Rate Transition/4(Out4) -> ctrlMode/1
  Control Rate Transition/5(Out5) -> FlightMode/1
  Ground/1 -> Guidance Logic/3(Ground)

== system EVTOLTiltrotor/Controls/Guidance Test Bench/ControlType/Manual Control ==
  Global Mission : Inport
  Aircraft States : Inport  Port=2
  Command Interface : Subsystem
  HoverCmds : Outport
  FixedWingSP : Outport  Port=2
  AACSP : Outport  Port=3
  ctrlMode : Outport  Port=4
  FlightMode : Outport  Port=5
  wires:
  Global Mission/1 -> Command Interface/1(Global Mission)
  Aircraft States/1 -> Command Interface/2(Aircraft States)
  Command Interface/1(ctrlMode) -> ctrlMode/1
  Command Interface/2(FixedWingSP) -> FixedWingSP/1
  Command Interface/3(AACSP) -> AACSP/1
  Command Interface/4(PositionCmds) -> HoverCmds/1
  Command Interface/5(FlightMode) -> FlightMode/1

== system EVTOLTiltrotor/Controls/Guidance Test Bench/Variant Subsystem/No-op ==
  State : Inport
  Terminator : Terminator
  wires:
  State/1 -> Terminator/1

== system EVTOLTiltrotor/Controls/Guidance Test Bench/Variant Subsystem/Reference Tracking  ==
  State : Inport
  Position : Inport  Port=2
  AAC : Inport  Port=3
  Fixed Wing Reference : Subsystem
  Hover Reference : Subsystem
  Transition Reference : Subsystem
  wires:
  State/1 -> Transition Reference/1(States), Fixed Wing Reference/2(States), Hover Reference/2(Position Reference)
  AAC/1 -> Fixed Wing Reference/1(AAC Commands)
  Position/1 -> Hover Reference/1(Position Command)

== system EVTOLTiltrotor/Controls/Output/Rotor Tilt/Tilt Servo Dynamics ==
  Rotor : Inport
  TiltB : Inport  Port=2
  Gain2 : Gain  Gain=pi/2
  Gain3 : Gain  Gain=pi/2
  IC : InitialCondition  Value=tiltIni
  IC1 : InitialCondition  Value=tiltIni
  Servo Dynamics : TransferFcn  Denominator=[0.1 1]
  Servo Dynamics1 : TransferFcn  Denominator=[0.1 1]
  Tilt1 : Outport
  Tilt2 : Outport  Port=2
  wires:
  Gain2/1 -> Servo Dynamics/1
  TiltB/1 -> Gain3/1
  Servo Dynamics/1 -> IC1/1
  Servo Dynamics1/1 -> IC/1
  IC/1 -> Tilt2/1  "Tilt2"
  IC1/1 -> Tilt1/1  "Tilt1"
  Gain3/1 -> Servo Dynamics1/1
  Rotor/1 -> Gain2/1

== system EVTOLTiltrotor/Controls/Guidance Test Bench/ControlType/Guidance Testbench/Control Rate Transition ==
  "1 " : Inport
  In2 : Inport  Port=2
  In3 : Inport  Port=3
  In4 : Inport  Port=4
  In5 : Inport  Port=5
  Rate Transition{,1..3} (4 alike) : RateTransition  OutPortSampleTime=ControlSampleTime
  Rate Transition4 : RateTransition  InitialCondition=flightState.Hover  OutPortSampleTime=ControlSampleTime
  Out1 : Outport
  Out2 : Outport  Port=2
  Out3 : Outport  Port=3
  Out4 : Outport  Port=4
  Out5 : Outport  Port=5
  wires:
  In4/1 -> Rate Transition3/1
  In2/1 -> Rate Transition1/1
  Rate Transition4/1 -> Out5/1
  In5/1 -> Rate Transition4/1
  Rate Transition3/1 -> Out4/1
  "1 "/1 -> Rate Transition/1
  Rate Transition1/1 -> Out2/1
  In3/1 -> Rate Transition2/1
  Rate Transition2/1 -> Out3/1
  Rate Transition/1 -> Out1/1

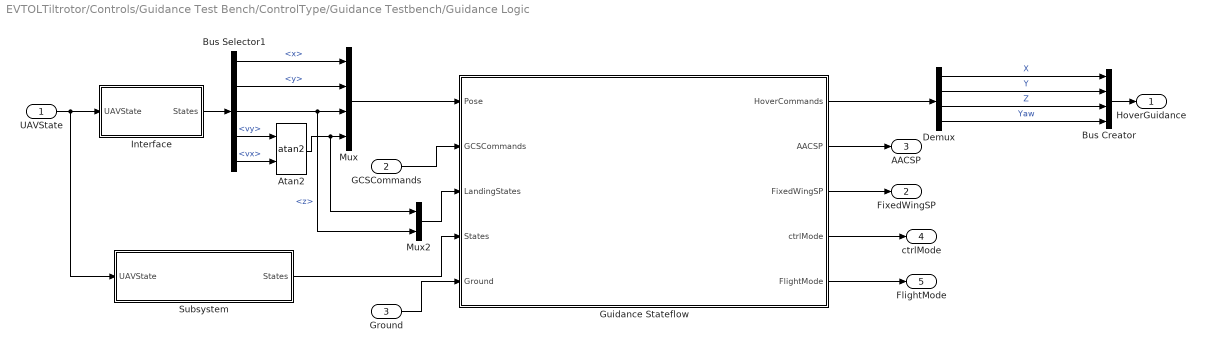
== system EVTOLTiltrotor/Controls/Guidance Test Bench/ControlType/Guidance Testbench/Guidance Logic ==
  UAVState : Inport
  GCSCommands : Inport  Port=2
  Ground : Inport  Port=3
  Atan2 : Trigonometry  Operator=atan2
  Bus Creator : BusCreator  Inputs=4
  Bus Selector1 : BusSelector  OutputSignals=x,y,z,vy,vx
  Demux : Demux
  Guidance Stateflow : Subsystem
  Interface : Subsystem
  Mux : Mux
  Mux2 : Mux  Inputs=2
  Subsystem : Subsystem
  HoverGuidance : Outport
  FixedWingSP : Outport  Port=2
  AACSP : Outport  Port=3
  ctrlMode : Outport  Port=4
  FlightMode : Outport  Port=5
  wires:
  Mux/1 -> Guidance Stateflow/1(Pose)
  Bus Selector1/5 -> Atan2/2  "<vx>"
  GCSCommands/1 -> Guidance Stateflow/2(GCSCommands)
  Bus Selector1/4 -> Atan2/1  "<vy>"
  Bus Selector1/3 -> Mux2/2, Mux/3  "<z>"
  Bus Selector1/2 -> Mux/2  "<y>"
  UAVState/1 -> Subsystem/1(UAVState), Interface/1(UAVState)
  Bus Selector1/1 -> Mux/1  "<x>"
  Guidance Stateflow/1(HoverCommands) -> Demux/1
  Interface/1(States) -> Bus Selector1/1
  Demux/3 -> Bus Creator/3  "Z"
  Demux/1 -> Bus Creator/1  "X"
  Demux/2 -> Bus Creator/2  "Y"
  Mux2/1 -> Guidance Stateflow/3(LandingStates)
  Atan2/1 -> Mux2/1, Mux/4
  Subsystem/1(States) -> Guidance Stateflow/4(States)
  Guidance Stateflow/3(FixedWingSP) -> FixedWingSP/1
  Guidance Stateflow/2(AACSP) -> AACSP/1
  Guidance Stateflow/4(ctrlMode) -> ctrlMode/1
  Guidance Stateflow/5(FlightMode) -> FlightMode/1
  Bus Creator/1 -> HoverGuidance/1
  Demux/4 -> Bus Creator/4  "Yaw"
  Ground/1 -> Guidance Stateflow/5(Ground)

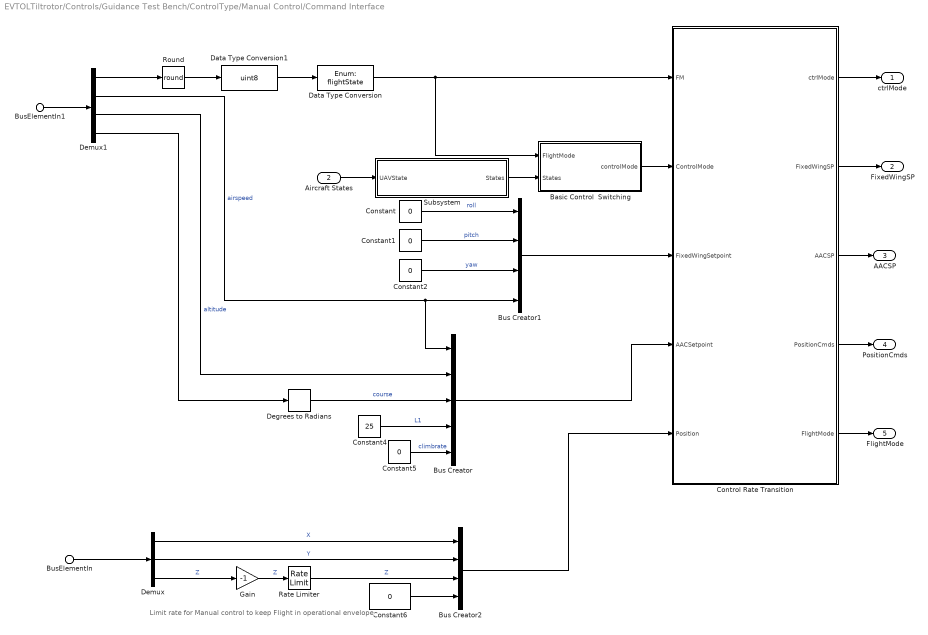
== system EVTOLTiltrotor/Controls/Guidance Test Bench/ControlType/Manual Control/Command Interface ==
  note: Limit rate for Manual control to keep Flight in operational envelope
  BusElementIn : Inport  PortName=Global Mission  Element=position
  BusElementIn1 : Inport  PortName=Global Mission  Element=params
  Aircraft States : Inport  Port=2
  Basic Control  Switching : Stateflow chart  TreatAsAtomicUnit=on
  Bus Creator : BusCreator  Inputs=5  OutDataTypeStr=Bus: AAC
  Bus Creator1 : BusCreator  Inputs=4  OutDataTypeStr=Bus: FixedWingCommandBus
  Bus Creator2 : BusCreator  Inputs=4
  Constant{,1..2,5..6} (5 alike) : Constant  Value=0
  Constant4 : Constant  Value=25
  Control Rate Transition : Subsystem
  Data Type Conversion : DataTypeConversion  OutDataTypeStr=Enum: flightState  SaturateOnIntegerOverflow=off  RndMeth=Floor
  Data Type Conversion1 : DataTypeConversion  OutDataTypeStr=uint8  SaturateOnIntegerOverflow=off  RndMeth=Floor
  Degrees to Radians : simulink_extras/Transformations/Degrees to Radians
  Demux : Demux  Outputs=3
  Demux1 : Demux
  Gain : Gain  Gain=-1
  Rate Limiter : RateLimiter  RisingSlewLimit=3  FallingSlewLimit=-3  SampleTimeMode=inherited
  Round : Rounding  Operator=round
  Subsystem : Subsystem
  ctrlMode : Outport
  FixedWingSP : Outport  Port=2
  AACSP : Outport  Port=3
  PositionCmds : Outport  Port=4
  FlightMode : Outport  Port=5
  wires:
  Demux1/3 -> Bus Creator/2  "altitude"
  Bus Creator2/1 -> Control Rate Transition/5(Position)
  Constant5/1 -> Bus Creator/5  "climbrate"
  Demux1/4 -> Degrees to Radians/1
  Bus Creator/1 -> Control Rate Transition/4(AACSetpoint)
  Demux/3 -> Gain/1  "Z"
  Data Type Conversion/1 -> Basic Control  Switching/1(FlightMode), Control Rate Transition/1(FM)
  Constant/1 -> Bus Creator1/1  "roll"
  Bus Creator1/1 -> Control Rate Transition/3(FixedWingSetpoint)
  Constant1/1 -> Bus Creator1/2  "pitch"
  Constant4/1 -> Bus Creator/4  "L1"
  Constant2/1 -> Bus Creator1/3  "yaw"
  Demux1/2 -> Bus Creator/1, Bus Creator1/4  "airspeed"
  Control Rate Transition/2(FixedWingSP) -> FixedWingSP/1
  Degrees to Radians/1 -> Bus Creator/3  "course"
  Demux/1 -> Bus Creator2/1  "X"
  Aircraft States/1 -> Subsystem/1(UAVState)
  Demux/2 -> Bus Creator2/2  "Y"
  Gain/1 -> Rate Limiter/1  "Z"
  Basic Control  Switching/1(controlMode) -> Control Rate Transition/2("ControlMode ")
  Control Rate Transition/1(ctrlMode) -> ctrlMode/1
  Control Rate Transition/3(AACSP) -> AACSP/1
  Control Rate Transition/4(PositionCmds) -> PositionCmds/1
  Control Rate Transition/5(FlightMode) -> FlightMode/1
  Demux1/1 -> Round/1
  Subsystem/1(States) -> Basic Control  Switching/2(States)
  Constant6/1 -> Bus Creator2/4
  Rate Limiter/1 -> Bus Creator2/3  "Z"
  BusElementIn/1 -> Demux/1
  BusElementIn1/1 -> Demux1/1
  Round/1 -> Data Type Conversion1/1
  Data Type Conversion1/1 -> Data Type Conversion/1

== system EVTOLTiltrotor/Controls/Guidance Test Bench/Variant Subsystem/Reference Tracking /Fixed Wing Reference ==
  AAC Commands : Inport
  States : Inport  Port=2
  Bus Creator1 : BusCreator  Inputs=2
  Bus Creator2 : BusCreator  Inputs=3
  Bus Selector : BusSelector  OutputSignals=airspeed,Xe,course
  Bus Selector3 : BusSelector  OutputSignals=airspeed,altitude,course
  Gain : Gain  Gain=-1
  Mux1 : Mux  Inputs=3
  Selector : Selector  InputPortWidth=3  IndexOptions=Index vector (dialog)  Indices=3  OutputSizes=1
  To Workspace1 : ToWorkspace  VariableName=FixedWingCmdFdbk  SaveFormat=Structure With Time  SampleTime=-1
  wires:
  Selector/1 -> Gain/1
  Bus Selector3/1 -> Mux1/1  "<airspeed>"
  Bus Selector/1 -> Bus Creator2/1  "<airspeed>"
  Bus Selector3/2 -> Mux1/2  "<altitude>"
  Bus Selector/3 -> Bus Creator2/3  "<course>"
  Mux1/1 -> Bus Creator1/1
  Bus Creator1/1 -> To Workspace1/1
  Bus Selector3/3 -> Mux1/3  "<course>"
  Gain/1 -> Bus Creator2/2  "altitude"
  Bus Creator2/1 -> Bus Creator1/2
  AAC Commands/1 -> Bus Selector3/1
  Bus Selector/2 -> Selector/1  "<Xe>"
  States/1 -> Bus Selector/1

== system EVTOLTiltrotor/Controls/Guidance Test Bench/Variant Subsystem/Reference Tracking /Hover Reference ==
  Position Command : Inport
  Position Reference : Inport  Port=2
  Bus Creator : BusCreator  Inputs=2
  Bus Selector1 : BusSelector  OutputSignals=Xe  OutputAsBus=on
  Bus Selector2 : BusSelector  OutputSignals=X,Y,Z
  Mux : Mux  Inputs=3
  To Workspace : ToWorkspace  VariableName=PositionCmdFdbk  SaveFormat=Structure With Time  SampleTime=-1
  wires:
  Position Reference/1 -> Bus Selector1/1
  Bus Selector2/3 -> Mux/3  "<Z>"
  Bus Selector2/1 -> Mux/1  "<X>"
  Bus Selector1/1 -> Bus Creator/2
  Bus Creator/1 -> To Workspace/1
  Bus Selector2/2 -> Mux/2  "<Y>"
  Mux/1 -> Bus Creator/1
  Position Command/1 -> Bus Selector2/1

== system EVTOLTiltrotor/Controls/Guidance Test Bench/Variant Subsystem/Reference Tracking /Transition Reference ==
  States : Inport
  Bus Creator : BusCreator  Inputs=4
  Bus Selector4 : BusSelector  OutputSignals=airspeed,RotorParameters.Tilt1,Euler,Xe
  Gain : Gain  Gain=-1
  Selector : Selector  InputPortWidth=3  IndexOptions=Index vector (dialog)  Indices=[2]  OutputSizes=1
  Selector1 : Selector  InputPortWidth=3  IndexOptions=Index vector (dialog)  Indices=[3]  OutputSizes=1
  To Workspace1 : ToWorkspace  VariableName=TransitionFeedback  SaveFormat=Structure With Time  SampleTime=-1
  wires:
  States/1 -> Bus Selector4/1
  Bus Selector4/3 -> Selector/1  "<Euler>"
  Bus Selector4/4 -> Selector1/1  "<Xe>"
  Selector1/1 -> Gain/1
  Bus Selector4/1 -> Bus Creator/1  "<airspeed>"
  Selector/1 -> Bus Creator/3  "pitch"
  Gain/1 -> Bus Creator/4  "altitude"
  Bus Creator/1 -> To Workspace1/1
  Bus Selector4/2 -> Bus Creator/2  "<Tilt1>"
